simulink model "acf_detector_sl"  (R2018b)
settings: Solver=VariableStepAuto  StartTime=0.0  StopTime=inf  RelTol=1e-3
model workspace (MAT data in the model file):
  SL_ROS_VariableLengthArrays_MaxSizes.CommonInfo.ArrayTruncateAction = 'EmitWarning'
  SL_ROS_VariableLengthArrays_MaxSizes.MsgTypeMap = containers.Map
  SL_ROS_VariableLengthArrays_MaxSizes.MsgTypeMap.serialization.keys = {'autoware_msgs/image_obj', 'sensor_msgs/Image'}
  SL_ROS_VariableLengthArrays_MaxSizes.MsgTypeMap.serialization.values{1}(1).PropertyName = 'Obj'
  SL_ROS_VariableLengthArrays_MaxSizes.MsgTypeMap.serialization.values{1}(1).DataType = 'autoware_msgs/image_rect'
  SL_ROS_VariableLengthArrays_MaxSizes.MsgTypeMap.serialization.values{1}(1).MaxLength = 16
  SL_ROS_VariableLengthArrays_MaxSizes.MsgTypeMap.serialization.values{1}(2).PropertyName = 'Type'
  SL_ROS_VariableLengthArrays_MaxSizes.MsgTypeMap.serialization.values{1}(2).DataType = 'uint8'
  SL_ROS_VariableLengthArrays_MaxSizes.MsgTypeMap.serialization.values{1}(2).MaxLength = 128
  SL_ROS_VariableLengthArrays_MaxSizes.MsgTypeMap.serialization.values{2}(1).PropertyName = 'Data'
  SL_ROS_VariableLengthArrays_MaxSizes.MsgTypeMap.serialization.values{2}(1).DataType = 'uint8'
  SL_ROS_VariableLengthArrays_MaxSizes.MsgTypeMap.serialization.values{2}(1).MaxLength = 1440000
  SL_ROS_VariableLengthArrays_MaxSizes.MsgTypeMap.serialization.values{2}(2).PropertyName = 'Encoding'
  SL_ROS_VariableLengthArrays_MaxSizes.MsgTypeMap.serialization.values{2}(2).DataType = 'uint8'
  SL_ROS_VariableLengthArrays_MaxSizes.MsgTypeMap.serialization.values{2}(2).MaxLength = 128
  SL_ROS_VariableLengthArrays_MaxSizes.MsgTypeMap.serialization.uniformity = 0
  SL_ROS_VariableLengthArrays_MaxSizes.MsgTypeMap.serialization.keyType = 'char'
  SL_ROS_VariableLengthArrays_MaxSizes.MsgTypeMap.serialization.valueType = 'any'
undefined symbols (not defined in the file): Header, Height, Obj, Obj_SL_Info, Score, Type, Type_SL_Info, Width, X, Y
libraries: robotlib x5
settings Model: Creator=handai  LastModifiedBy=handai
settings DebuggingCC: LibraryContextMissingDiagnostic=none
settings SFSimCC: SimUseLocalCustomCode=off
settings RTWCC: RTWUseLocalCustomCode=off

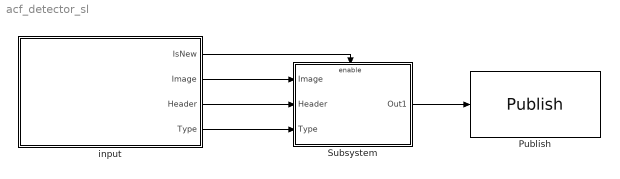
== system acf_detector_sl ==
  Publish : robotlib/Publish  topicSource=Specify your own  topic=/obj_person/image_obj  messageType=autoware_msgs/image_obj  messageQueueLength=1
      settings: SourceProductBaseCode=RO
  Subsystem : Subsystem
  input : Subsystem
  wires:
  input/1(IsNew) -> Subsystem/Enable
  input/2(Image) -> Subsystem/1(Image)
  input/3(Header) -> Subsystem/2(Header)
  input/4(Type) -> Subsystem/3(Type)
  Subsystem/1(Out1) -> Publish/1

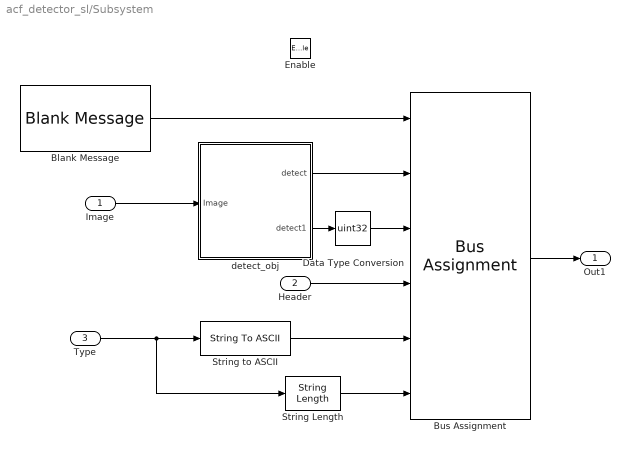
== system acf_detector_sl/Subsystem ==
  Image : Inport
  Header : Inport  Port=2
  Type : Inport  Port=3
  Enable : EnablePort  PropagateVarSize=During execution
  Blank Message : robotlib/Blank Message  messageClass=Message  entityType=autoware_msgs/image_obj  messageType=autoware_msgs/image_obj  SampleTime=inf
      settings: SourceProductBaseCode=RO
  Bus Assignment : BusAssignment  AssignedSignals=Obj,Obj_SL_Info.CurrentLength,Header,Type,Type_SL_Info.CurrentLength
  Data Type Conversion : DataTypeConversion  OutDataTypeStr=uint32
  String Length : StringLength
  String to ASCII : StringToASCII  MaximumLength=128
  detect_obj : Subsystem
  Out1 : Outport
  wires:
  Bus Assignment/1 -> Out1/1
  Type/1 -> String Length/1, String to ASCII/1
  Image/1 -> detect_obj/1(Image)
  Blank Message/1 -> Bus Assignment/1
  detect_obj/1(detect) -> Bus Assignment/2
  Header/1 -> Bus Assignment/4
  String to ASCII/1 -> Bus Assignment/5
  String Length/1 -> Bus Assignment/6
  detect_obj/2(detect1) -> Data Type Conversion/1
  Data Type Conversion/1 -> Bus Assignment/3

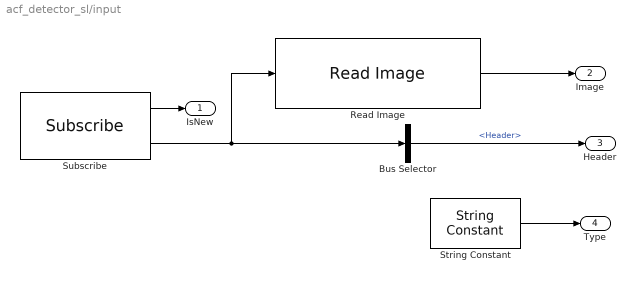
== system acf_detector_sl/input ==
  Bus Selector : BusSelector  OutputSignals=Header
  Read Image : robotlib/Read Image  MaximumImageSize=[ 2000 1800 ]  ImageEncoding=rgb8  ShowAlphaOutput=off  ShowErrorCodeOutput=off  VariableSizeOutputs=off
      settings: SourceProductName=Robotics System Toolbox  SourceProductBaseCode=RO
  String Constant : StringConstant  String='Person'
  Subscribe : robotlib/Subscribe  topicSource=Specify your own  topic=/image_raw  messageType=sensor_msgs/Image  sampleTime=-1  messageQueueLength=1
      settings: SourceProductBaseCode=RO
  IsNew : Outport
  Image : Outport  Port=2
  Header : Outport  Port=3
  Type : Outport  Port=4
  wires:
  Read Image/1 -> Image/1
  String Constant/1 -> Type/1
  Bus Selector/1 -> Header/1  "<Header>"
  Subscribe/1 -> IsNew/1
  Subscribe/2 -> Read Image/1, Bus Selector/1

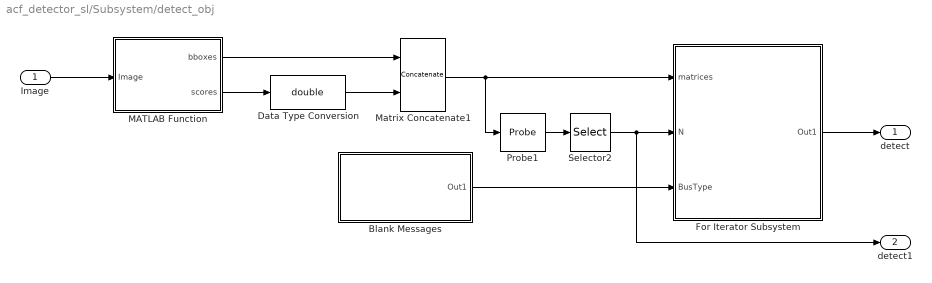
== system acf_detector_sl/Subsystem/detect_obj ==
  Image : Inport
  Blank Messages : Subsystem
  Data Type Conversion : DataTypeConversion  OutDataTypeStr=double
  For Iterator Subsystem : Subsystem  TreatAsAtomicUnit=on
  MATLAB Function : MATLAB Function  TreatAsAtomicUnit=on
  Matrix Concatenate1 : Concatenate  Mode=Multidimensional array  ConcatenateDimension=2
  Probe1 : Probe  ProbeWidth=off  ProbeSampleTime=off  ProbeComplexSignal=off  ProbeSignalDimensions=on
  Selector2 : Selector  InputPortWidth=2  IndexOptions=Index vector (dialog)  Indices=1  OutputSizes=1
  detect : Outport
  detect1 : Outport  Port=2
  wires:
  Image/1 -> MATLAB Function/1(Image)
  MATLAB Function/1(bboxes) -> Matrix Concatenate1/1
  MATLAB Function/2(scores) -> Data Type Conversion/1
  Data Type Conversion/1 -> Matrix Concatenate1/2
  For Iterator Subsystem/1(Out1) -> detect/1
  Blank Messages/1(Out1) -> For Iterator Subsystem/3(BusType)
  Matrix Concatenate1/1 -> Probe1/1, For Iterator Subsystem/1(matrices)
  Selector2/1 -> For Iterator Subsystem/2(N), detect1/1
  Probe1/1 -> Selector2/1

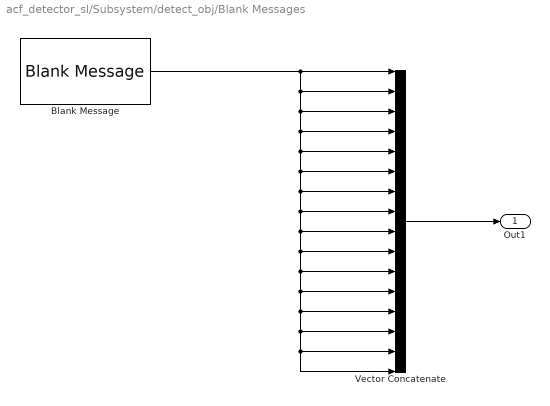
== system acf_detector_sl/Subsystem/detect_obj/Blank Messages ==
  Blank Message : robotlib/Blank Message  messageClass=Message  entityType=autoware_msgs/image_rect  messageType=autoware_msgs/image_rect  SampleTime=inf
      settings: SourceProductBaseCode=RO
  Vector Concatenate : Concatenate  NumInputs=16
  Out1 : Outport
  wires:
  Blank Message/1 -> Vector Concatenate/4, Vector Concatenate/6, Vector Concatenate/12, Vector Concatenate/16, Vector Concatenate/15, Vector Concatenate/14, Vector Concatenate/13, Vector Concatenate/11, Vector Concatenate/10, Vector Concatenate/9, Vector Concatenate/8, Vector Concatenate/7, Vector Concatenate/5, Vector Concatenate/3, Vector Concatenate/2, Vector Concatenate/1
  Vector Concatenate/1 -> Out1/1

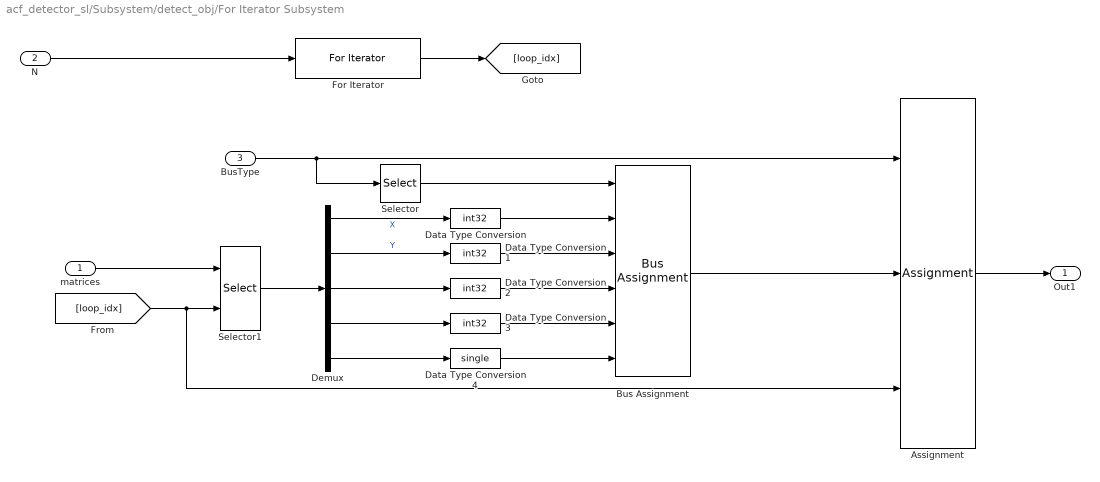
== system acf_detector_sl/Subsystem/detect_obj/For Iterator Subsystem ==
  matrices : Inport
  N : Inport  Port=2
  BusType : Inport  Port=3
  Assignment : Assignment  DiagnosticForDimensions=Warning  IndexOptions=Index vector (port)  Indices=1  OutputSizes=1
  Bus Assignment : BusAssignment  AssignedSignals=X,Y,Width,Height,Score
  Data Type Conversion{,1..3} (4 alike) : DataTypeConversion  OutDataTypeStr=int32
  Data Type Conversion4 : DataTypeConversion  OutDataTypeStr=single
  Demux : Demux  Outputs=5
  For Iterator : ForIterator  ResetStates=reset  IterationSource=external
  Selector : Selector  InputPortWidth=16  IndexOptions=Index vector (dialog)  Indices=1  OutputSizes=1
  Selector1 : Selector  NumberOfDimensions=2  IndexOptions=Index vector (port),Index vector (dialog)  Indices=1,[1:5]  OutputSizes=1,1
  Out1 : Outport
  wires:
  Assignment/1 -> Out1/1
  BusType/1 -> Selector/1, Assignment/1
  Selector1/1 -> Demux/1
  matrices/1 -> Selector1/1
  For Iterator/1 -> [loop_idx]
  [loop_idx] -> Assignment/3, Selector1/2
  N/1 -> For Iterator/1
  Selector/1 -> Bus Assignment/1
  Demux/3 -> Data Type Conversion2/1
  Demux/2 -> Data Type Conversion1/1  "Y"
  Demux/1 -> Data Type Conversion/1  "X"
  Demux/4 -> Data Type Conversion3/1
  Demux/5 -> Data Type Conversion4/1
  Data Type Conversion/1 -> Bus Assignment/2
  Data Type Conversion1/1 -> Bus Assignment/3
  Data Type Conversion2/1 -> Bus Assignment/4
  Data Type Conversion3/1 -> Bus Assignment/5
  Data Type Conversion4/1 -> Bus Assignment/6
  Bus Assignment/1 -> Assignment/2

== matlab function acf_detector_sl/Subsystem/detect_obj/MATLAB Function ==
  settings: updateMethod=DISCRETE
  data: Image input; bboxes output size=[16 4]; scores output size=[16 1]
function [bboxes, scores] = fcn(Image)
    coder.extrinsic('detectPeopleACF');
    bboxes = zeros(16, 4);
    scores = zeros(16, 1);
[bboxes, scores] = detectPeopleACF(Image);
